simulink library "sf_elevator_lib"  (R2021b)
settings: Solver=FixedStepDiscrete  StartTime=0.0  StopTime=10.0  FixedStep=1  RelTol=1e-3  EnableMultiTasking=on
settings Model: Creator=The MathWorks, Inc.  LastModifiedBy=The MathWorks, Inc.
settings SolverCC: AlgebraicLoopSolver=TrustRegion
settings DataIOCC: LimitDataPoints=on  SaveFormat=Array  SignalLoggingSaveFormat=ModelDataLogs  ReturnWorkspaceOutputs=off
settings OptimizationCC: ExpressionDepthLimit=2147483647  LifeSpan=inf
settings DebuggingCC: UnderspecifiedInitializationDetection=Classic  MergeDetectMultiDrivingBlocksExec=none  SolverPrmCheckMsg=warning  FcnCallInpInsideContextMsg=warning  StateNameClashWarn=warning  SFUnexpectedBacktrackingDiag=warning  SFNoUnconditionalDefaultTransitionDiag=warning  SFExecutionAtInitializationDiag=none  SFMachineParentedDataDiag=warning  ArithmeticOperatorsInVariantConditions=warning
settings HardwareCC: ProdBitPerPointer=32  ProdBitPerSizeT=32  ProdBitPerPtrDiffT=32  ProdLargestAtomicFloat=None  ProdIntDivRoundTo=Undefined  ProdEndianess=Unspecified  ProdWordSize=32  ProdHWDeviceType=32-bit Generic
settings ModelReferenceCC: PropagateSignalLabelsOutOfModel=off
settings SFSimCC: SimUseLocalCustomCode=off  CustomCodeUndefinedFunction=UseInterfaceOnly
settings RTWCC: RTWUseLocalCustomCode=off
settings CodeAppCC: StateflowObjectComments=on
settings GRTTargetCC: TargetLangStandard=C89/C90 (ANSI)  CombineOutputUpdateFcns=off  GRTInterface=on
settings ConfigComp: CovMetricSettings=dw  CovSaveCumulativeToWorkspaceVar=on  CovSaveSingleToWorkspaceVar=on  CovExternalEMLEnable=off  CovSFcnEnable=off

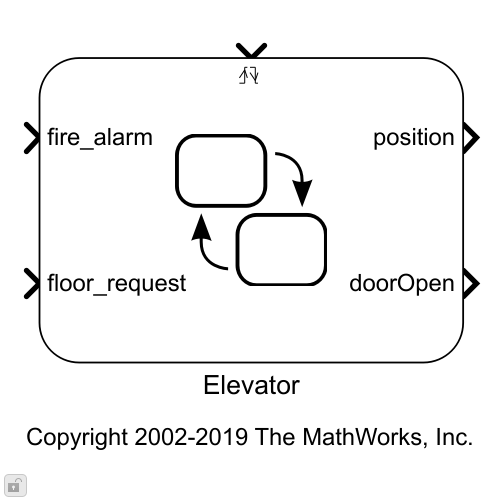
[thumbnail: Simulink's stored preview of the top-level diagram]
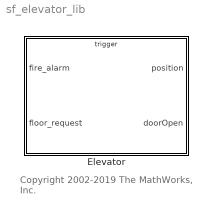
== system sf_elevator_lib ==
  note: Copyright 2002-2019 The MathWorks, Inc.
  Elevator : Stateflow chart  TreatAsAtomicUnit=on

== stateflow chart sf_elevator_lib/Elevator ==
  state Elevator
    state PickUpDropOff
      en: Main_deregister(cur_floor);
      deregister(cur_floor);
      direction = MOVE_IDLE;
      doorOpen = 1;
      du: Main_deregister(cur_floor);
      deregister(cur_floor);
      ex: doorOpen = 0;
      state Stopped
      Stopped -> Stopped [order 1] : [fire_alarm]{status = EMERG;
          | resetTheElevatorCar();}
          | /* Resets the timeout counter */
    state Idle
      en: status = IDLE;
      ex: status = BUSY;
    state MoveToTask
      du: move_to(task_queue[0]);
    Elevator -> (junction 789) : CAR_CALL  {register(floor_request);}
    (default) -> Idle : {doorOpen = 0;}
    (junction 8) -> Idle [order 2]
    Stopped -> (junction 8) [order 2] : after(TIME_OUT, CLOCK)
    (junction 8) -> MoveToTask [order 1] : [task_queue[0]]
    Idle -> MoveToTask : [task_queue[0]]
    MoveToTask -> PickUpDropOff : [should_stop()]
  state ans = should_stop [function]
    (default) -> (junction 982)
    (junction 982) -> (junction 984) : {
        | /* 'INIT':Initialization */
        | cur_floor = ml_round(position);
        | }
    (junction 984) -> (junction 986) : {
        | /* Fire Alarm */
        | fire_alarm_on = (fire_alarm);
        | }
    (junction 986) -> (junction 988) : {
        | /* Arrived destination */
        | at_destination = (fabs(position - task_queue[0]) < ERR_TOR);
        | }
    (junction 988) -> (junction 990) : {
        | /* Arrived at a floor */
        | at_a_floor = (fabs(position - cur_floor) < ERR_TOR);
        | }
    (junction 990) -> (junction 992) : {
        | /* There is car call to stop at this floor */
        | request_from_car = (car_call_status[cur_floor]);
        | }
    (junction 992) -> (junction 994) : {
        | /* There is hall call from this floor */
        | request_from_hall = (hall_call_status[cur_floor]);
        | }
    (junction 994) -> (junction 996) : {
        | /* This hall call is still outstanding in queue */
        | this_hall_call_outstanding = (Main_exists_in_queue(cur_floor));
        | }
    (junction 996) -> (junction 998) [order 1] : [fire_alarm_on]
    (junction 998) -> (junction 1000) : {
        | /* 'S':Should stop at this floor */
        | position = cur_floor; /* Adjust position */
        | ans = 1;
        | }
    (junction 996) -> (junction 1002) [order 2]
    (junction 1002) -> (junction 1004) [order 1] : [at_destination]
    (junction 1004) -> (junction 1006) : {
        | /* 'S':Should stop at this floor */
        | position = cur_floor; /* Adjust position */
        | ans = 1;
        | }
    (junction 1002) -> (junction 1008) [order 2]
    (junction 1008) -> (junction 1010) [order 1] : [!at_a_floor]
    (junction 1010) -> (junction 1012) : {
        | /* 'C':Should not stop, continue */
        | ans = 0;
        | }
    (junction 1008) -> (junction 1014) [order 2]
    (junction 1014) -> (junction 1016) [order 1] : [request_from_car]
    (junction 1016) -> (junction 1018) : {
        | /* 'S':Should stop at this floor */
        | position = cur_floor; /* Adjust position */
        | ans = 1;
        | }
    (junction 1014) -> (junction 1020) [order 2]
    (junction 1020) -> (junction 1022) [order 1] : [request_from_hall && this_hall_call_outstanding]
    (junction 1022) -> (junction 1024) : {
        | /* 'S':Should stop at this floor */
        | position = cur_floor; /* Adjust position */
        | ans = 1;
        | }
    (junction 1020) -> (junction 1026) [order 2]
    (junction 1026) -> (junction 1028) : /* Default */
    (junction 1028) -> (junction 1030) : {
        | /* 'C':Should not stop, continue */
        | ans = 0;
        | }
  state move_to(destination) [function]
    (default) -> (junction 1034)
    (junction 1034) -> (junction 1036) : {
        | /* Move up */
        | move_up = (destination - position > ERR_TOR);
        | }
    (junction 1036) -> (junction 1038) : {
        | /* Move down */
        | move_down = (position - destination > ERR_TOR);
        | }
    (junction 1038) -> (junction 1040) [order 1] : [move_up && !move_down]
    (junction 1040) -> (junction 1042) : {
        | /* Move up */
        | position = position + VELOCITY;
        | direction = MOVE_UP;
        | }
    (junction 1038) -> (junction 1044) [order 2]
    (junction 1044) -> (junction 1046) : [!move_up && move_down]
    (junction 1046) -> (junction 1048) : {
        | /* Move down */
        | position = position - VELOCITY;
        | direction = MOVE_DOWN;
        | }
  state dir = get_direction [function]
    (default) -> (junction 93) : {dir = direction;}
  state enqueue(task_floor) [function]
    (default) -> (junction 102)
    (junction 102) -> (junction 103) [order 1] : [car_call_status[task_floor] != 0]
    (junction 102) -> (junction 105) [order 2] : {i = 0;}
    (junction 105) -> (junction 104) [order 1] : [task_queue[i] == task_floor]
    (junction 105) -> (junction 105) [order 2] : [task_queue[i] > 0 && i<NUM_FLOOR]{i++;}
    (junction 105) -> (junction 106) [order 3]
    (junction 106) -> (junction 107) [order 1] : [i >= NUM_FLOOR]
    (junction 106) -> (junction 108) [order 2] : {task_queue[i] = task_floor;}
  state register(car_call_floor) [function]
    (default) -> (junction 719) : {enqueue(car_call_floor);
        | car_call_status[car_call_floor] = 1;}
  state pos = get_position [function]
    (default) -> (junction 119) : {pos = position;}
  state dequeue(task_floor) [function]
    (default) -> (junction 132) : {i=0;}
    (junction 132) -> (junction 132) [order 1] : [task_queue[i] > 0 && ...
        | i<NUM_FLOOR && ...
        | task_queue[i] != task_floor]{i++;}
    (junction 132) -> (junction 133) [order 2]
    (junction 133) -> (junction 134) [order 1] : [i >= NUM_FLOOR || task_queue[i] == 0]
    (junction 133) -> (junction 135) [order 2]
    (junction 135) -> (junction 136) : {task_queue[i] = task_queue[i+1]; i++;}
    (junction 136) -> (junction 135) [order 1] : [i < NUM_FLOOR]
    (junction 136) -> (junction 137) [order 2]
  state deregister(car_call_floor) [function]
    (default) -> (junction 123) : {dequeue(car_call_floor);
        | car_call_status[car_call_floor] = 0;}
  state stat = get_status [function]
    (default) -> (junction 127) : {stat = status;}
  state resetTheElevatorCar [function]
    (default) -> (junction 856) : /* deregister every floor */
    (junction 855) -> (junction 853) [order 1] : [i<NUM_FLOOR]
    (junction 853) -> (junction 854) : {deregister(i+1);
        | Main_deregister(i+1);
        | ml.sf_elevator_gui('deactivate', 'hall', i+1);
        | ml.sf_elevator_gui('deactivate', 1, (i+1));
        | ml.sf_elevator_gui('deactivate', 2, (i+1));}
    (junction 856) -> (junction 855) : {i=0;}
    (junction 854) -> (junction 855) : {i++;}
    (junction 855) -> (junction 852) [order 2]
  data: ans function_output boolean; fire_alarm_on temporary boolean =0; at_destination temporary boolean =0; at_a_floor temporary boolean =0; request_from_car temporary boolean =0; request_from_hall temporary boolean =0; this_hall_call_outstanding temporary boolean =0; destination function_input double; move_up temporary boolean =0; move_down temporary boolean =0; dir function_output uint8; task_floor function_input uint8; i temporary uint8; car_call_floor function_input uint8; pos function_output double; i temporary uint8; task_floor function_input uint8; car_call_floor function_input uint8; stat function_output uint8; inputVal function_input double; out function_output double; i temporary uint8; VELOCITY constant double =0.005; NUM_FLOOR constant uint8 =9; ERR_TOR constant double =0.001; fire_alarm input boolean; TIME_OUT constant uint32 =1000; status local Enum: ElevatorStatus =ElevatorStatus.IDLE; position output double =1; task_queue local uint8 size=10; car_call_status local uint8 size=10; direction local Enum: ElevatorDirection =ElevatorDirection.MOVE_IDLE; doorOpen output boolean; cur_floor local uint8; hall_call_status data_store_memory; floor_request input
  data fire_alarm_on settings: description=Fire Alarm
  data at_destination settings: description=Arrived destination
  data at_a_floor settings: description=Arrived at a floor
  data request_from_car settings: description=There is car call to stop at this floor
  data request_from_hall settings: description=There is hall call from this floor
  data this_hall_call_outstanding settings: description=This hall call is still outstanding in queue
  data move_up settings: description=Move up
  data move_down settings: description=Move down
  events: CAR_CALL input EITHER_EDGE_EVENT; CLOCK input EITHER_EDGE_EVENT
  function out = ml_round(inputVal):
    | function out = ml_round(inputVal)
    | 
    | out = round(inputVal);
